simulink model "usability"  (R2023b)
settings: Solver=FixedStepAuto  StartTime=0.0  StopTime=11  FixedStep=1  RelTol=1e-3
libraries: sensors_subsystems x1
settings Model: Creator=brent  LastModifiedBy=brent

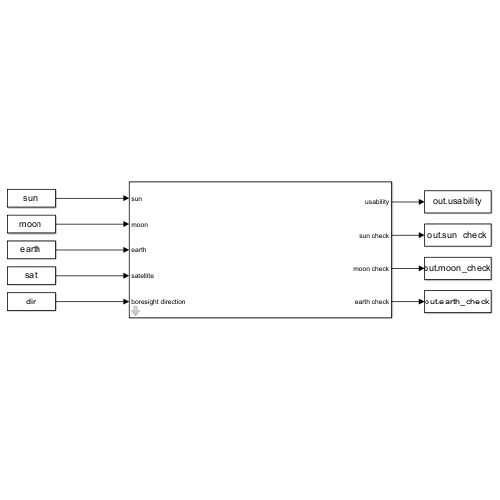
[thumbnail: Simulink's stored preview of the top-level diagram]
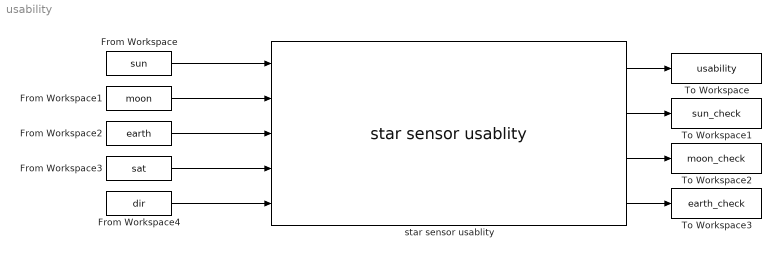
== system usability ==
  From Workspace : FromWorkspace  VariableName=sun
  From Workspace1 : FromWorkspace  VariableName=moon
  From Workspace2 : FromWorkspace  VariableName=earth
  From Workspace3 : FromWorkspace  VariableName=sat
  From Workspace4 : FromWorkspace  VariableName=dir
  To Workspace : ToWorkspace  VariableName=usability  SaveFormat=Timeseries  SampleTime=-1
  To Workspace1 : ToWorkspace  VariableName=sun_check  SaveFormat=Timeseries  SampleTime=-1
  To Workspace2 : ToWorkspace  VariableName=moon_check  SaveFormat=Timeseries  SampleTime=-1
  To Workspace3 : ToWorkspace  VariableName=earth_check  SaveFormat=Timeseries  SampleTime=-1
  star sensor usablity : sensors_subsystems/star sensor usablity  R_M=R_M  R_E=R_E  exclusionAngle=exclusionAngle  fov=fov
      settings: SourceProductName=Sensors library
  wires:
  From Workspace/1 -> star sensor usablity/1
  From Workspace1/1 -> star sensor usablity/2
  From Workspace2/1 -> star sensor usablity/3
  From Workspace3/1 -> star sensor usablity/4
  From Workspace4/1 -> star sensor usablity/5
  star sensor usablity/1 -> To Workspace/1
  star sensor usablity/2 -> To Workspace1/1
  star sensor usablity/3 -> To Workspace2/1
  star sensor usablity/4 -> To Workspace3/1
